simulink model "torqueBalancingTuning"  (Simulink 8.7)
settings: Solver=FixedStepDiscrete  StartTime=0.0  StopTime="CONFIG.SIMULATION_TIME "  FixedStep=CONFIG.Ts  RelTol=1e-3
InitFcn:
  | cd(fileparts(which(bdroot)));
  | initTorqueBalancing;
values from neighbouring files (symbols this model uses):
  baseToWorldRotationPort = ['/' WBT_modelName '/floatingBaseRotationMatrix:i']    [initTorqueBalancing.m]
  WBT_modelName = 'matlabTorqueBalancing'    [initTorqueBalancing.m]
undefined symbols (not defined in the file or in its folder): bVectorConstraints, CONFIG, ConstraintsMatrix, DiscIntNeverNeededParam, gain, references, reg, ROBOT_DOF, ROBOT_DOF_FOR_SIMULINK, sat, SM, sm, WBT_robotName
libraries: WBToolboxLibrary x171, simulink x11
(part 2 of 4)

== system torqueBalancingTuning/DesValues/Subsystem ==
  conn status 1 : Inport
  conn status 2 : Inport  Port=2
  conn status 3 : Inport  Port=3
  Compare To Zero3 : simulink/Logic and Bit Operations/Compare To Zero  relop=>  OutDataTypeStr=boolean
  Compare To Zero4 : simulink/Logic and Bit Operations/Compare To Zero  relop=>  OutDataTypeStr=boolean
  Compare To Zero5 : simulink/Logic and Bit Operations/Compare To Zero  relop=>  OutDataTypeStr=boolean
  Logical Operator : Logic  Inputs=3  AllPortsSameDT=off  OutDataTypeStr=boolean
  connection check : Outport
  wires:
  Logical Operator/1 -> connection check/1
  Compare To Zero4/1 -> Logical Operator/3
  conn status 1/1 -> Compare To Zero3/1
  Compare To Zero3/1 -> Logical Operator/1
  conn status 3/1 -> Compare To Zero4/1
  Compare To Zero5/1 -> Logical Operator/2
  conn status 2/1 -> Compare To Zero5/1

== system torqueBalancingTuning/Dump and visualize/ZMPs ==
  fDesQP : Inport
  Demux1 : Demux  Outputs=3
  Demux2 : Demux  Outputs=3
  Divide{4..7} (4 alike) : Product  Inputs=*/
  Gain3 : Gain  Gain=-1
  Gain4 : Gain  Gain=-1
  Mux : Mux  Inputs=2
  Mux1 : Mux  Inputs=2
  fz taux tauy Left : Selector  InputPortWidth=12  IndexOptions=Index vector (dialog)  Indices=[3 4 5]  OutputSizes=1
  fz taux tauy Right : Selector  InputPortWidth=12  IndexOptions=Index vector (dialog)  Indices=[9 10 11]  OutputSizes=1
  ZMP_LeftFoot : Outport
  ZMP_RightFoot : Outport  Port=2
  wires:
  fz taux tauy Left/1 -> Demux1/1
  Demux1/1 -> Divide4/2, Divide5/2
  Divide7/1 -> Gain4/1
  Divide4/1 -> Mux/2
  Divide5/1 -> Gain3/1
  fz taux tauy Right/1 -> Demux2/1
  Demux2/1 -> Divide6/2, Divide7/2
  fDesQP/1 -> fz taux tauy Left/1, fz taux tauy Right/1
  Gain3/1 -> Mux/1
  Mux/1 -> ZMP_LeftFoot/1
  Divide6/1 -> Mux1/2
  Gain4/1 -> Mux1/1
  Mux1/1 -> ZMP_RightFoot/1
  Demux1/2 -> Divide4/1  "tauxL"
  Demux1/3 -> Divide5/1  "tauyL"
  Demux2/2 -> Divide6/1  "tauxR"
  Demux2/3 -> Divide7/1  "tauyR"

== system torqueBalancingTuning/Dump and visualize/plotNorms ==
  qTile_LeftLeg : Inport
  qTile_RightLeg : Inport  Port=2
  state : Inport  Port=3
  Constant : Constant  Value=sm.joints.thresholdInContact
  Constant2 : Constant  Value=sm.joints.thresholdNotInContact
  Mux : Mux  Inputs=3
  Mux1 : Mux  Inputs=3
  norm : MATLAB Function  TreatAsAtomicUnit=on
  norm(qTilde) : Scope  NumInputPorts=3
  norm1 : MATLAB Function  TreatAsAtomicUnit=on
  wires:
  Constant/1 -> Mux1/2, Mux/2  "thresholdInContact"
  qTile_LeftLeg/1 -> norm1/1(u)
  qTile_RightLeg/1 -> norm/1(u)
  norm/1(normU) -> Mux1/1  "norm(qTilde_RightL)"
  norm1/1(normU) -> Mux/1  "norm(qTilde_LeftL)"
  Mux/1 -> norm(qTilde)/1
  Mux1/1 -> norm(qTilde)/2
  Constant2/1 -> Mux1/3, Mux/3  "thresholdNotInContact"
  state/1 -> norm(qTilde)/3

== system torqueBalancingTuning/controller_QP/QP ==
  LEFT_RIGHT_FOOT_IN_CONTACT : Inport
  HessianMatrixQP1Foot : Inport  Port=2
  gradientQP1Foot : Inport  Port=3
  ConstraintsMatrixQP1Foot : Inport  Port=4
  bVectorConstraintsQP1Foot : Inport  Port=5
  HessianMatrixQP2Feet : Inport  Port=6
  gradientQP2Feet : Inport  Port=7
  ConstraintsMatrixQP2Feet : Inport  Port=8
  bVectorConstraintsQp2Feet : Inport  Port=9
  state : Inport  Port=10
  Constant1 : Constant  Value=CONFIG.USE_QP_SOLVER
  Level-2 MATLAB S-Function : M-S-Function  FunctionName=QpBalancing
  Logical Operator1 : Logic  Operator=OR  AllPortsSameDT=off  OutDataTypeStr=boolean
  ON_GAZEBO 3 : Constant  Value=CONFIG.SCOPES.ALL
  ON_GAZEBO 4 : Constant  Value=CONFIG.SCOPES.QP
  QP two feet fails : Assertion  Commented=on
  Visualize eventual QP failures : Subsystem
  f0OneFoot : Outport
  f0TwoFeet : Outport  Port=2
  wires:
  Level-2 MATLAB S-Function/1 -> f0TwoFeet/1
  Level-2 MATLAB S-Function/2 -> Visualize eventual QP failures/1(exitFlagQP), QP two feet fails/1  "Exit flag QP two feet"
  HessianMatrixQP1Foot/1 -> Level-2 MATLAB S-Function/7
  gradientQP1Foot/1 -> Level-2 MATLAB S-Function/8
  ConstraintsMatrixQP1Foot/1 -> Level-2 MATLAB S-Function/9
  bVectorConstraintsQP1Foot/1 -> Level-2 MATLAB S-Function/10
  Level-2 MATLAB S-Function/3 -> f0OneFoot/1
  Logical Operator1/1 -> Visualize eventual QP failures/Enable
  state/1 -> Visualize eventual QP failures/2(state)
  LEFT_RIGHT_FOOT_IN_CONTACT/1 -> Level-2 MATLAB S-Function/1
  HessianMatrixQP2Feet/1 -> Level-2 MATLAB S-Function/2
  gradientQP2Feet/1 -> Level-2 MATLAB S-Function/3
  ConstraintsMatrixQP2Feet/1 -> Level-2 MATLAB S-Function/4
  bVectorConstraintsQp2Feet/1 -> Level-2 MATLAB S-Function/5
  Constant1/1 -> Level-2 MATLAB S-Function/6
  ON_GAZEBO 3/1 -> Logical Operator1/1
  ON_GAZEBO 4/1 -> Logical Operator1/2

== system torqueBalancingTuning/controller_QP/integralOf Hw1 ==
  qjDes : Inport
  qj : Inport  Port=2
  constraints : Inport  Port=3
  Centroidal Momentum : WBToolboxLibrary/wholeBodyModel/Dynamics/Centroidal Momentum  robotName=WBT_robotName  localName=WBT_modelName  wbiFile=WBT_wbiFilename  wbiList=WBT_wbiList
  Jacobian : WBToolboxLibrary/wholeBodyModel/Jacobians/Jacobian  frameName='l_sole'  robotName=WBT_robotName  localName=WBT_modelName  wbiFile=WBT_wbiFilename  wbiList=WBT_wbiList
  Jacobian1 : WBToolboxLibrary/wholeBodyModel/Jacobians/Jacobian  frameName='r_sole'  robotName=WBT_robotName  localName=WBT_modelName  wbiFile=WBT_wbiFilename  wbiList=WBT_wbiList
  MATLAB Function : MATLAB Function  TreatAsAtomicUnit=on
  Selector : Selector  InputPortWidth=6  IndexOptions=Index vector (dialog)  Indices=[4 5 6]  OutputSizes=1
  Sum : Sum  Inputs=|-+
  inertial : WBToolboxLibrary/Utilities/Yarp Read  portName=PORTS.IMU  signalSize=12  blocking=off  timestamp=off  autoconnect=on  errorOnConnection=on
  w_H_root_link4 : Subsystem  mask{link_name='l_sole'}
      mask prompts: link_name "link name"
      mask help:
      | This block evaluates the homogeneous transformation between the world and the root link, i.e. ^wH_b. It assumes that the link specified by the variable 'link_name' has a constant position
      | w.r.t. an inertial frame, but it can rotate arbitrarily. This rotation is retrived from the IMU sensor.
      mask Display:
      | str = strrep(link_name, '_','\_');
      | port_label('output',1,['{}^{',str '}H_{root}'],'texmode','on')
      | clear str;
      | 
      | port_label('input',1,'q_j','texmode','on')
      | 
      | port_label('input',2,'inertial','texmode','on')
  intHw : Outport
  wires:
  qjDes/1 -> Sum/1, Jacobian1/2, Jacobian/2, Centroidal Momentum/2, w_H_root_link4/1(qj)
  w_H_root_link4/1(w_H_root) -> Centroidal Momentum/1, Jacobian/1, Jacobian1/1
  qj/1 -> Sum/2
  Sum/1 -> Centroidal Momentum/4, MATLAB Function/1(qjErr)
  MATLAB Function/1(vbEquivalent) -> Centroidal Momentum/3
  Jacobian/1 -> MATLAB Function/2(JL)
  Centroidal Momentum/1 -> Selector/1
  Selector/1 -> intHw/1
  Jacobian1/1 -> MATLAB Function/3(JR)
  constraints/1 -> MATLAB Function/4(activeFeetConstraints)
  inertial/1 -> w_H_root_link4/2(inertial)

== system torqueBalancingTuning/controller_QP/xCom ==
  w_H_b : Inport
  qj : Inport  Port=2
  "CoM6D ->  CoMXYZ2" : Selector  NumberOfDimensions=2  InputPortWidth=7  IndexOptions=Index vector (dialog),Index vector (dialog)  Indices=[1 2 3],[4]  OutputSizes=1,1
  com : WBToolboxLibrary/wholeBodyModel/Kinematics/Forward Kinematics  frameName='com'  robotName=WBT_robotName  localName=WBT_modelName  wbiFile=WBT_wbiFilename  wbiList=WBT_wbiList
  xCom : Outport
  wires:
  qj/1 -> com/2
  "CoM6D ->  CoMXYZ2"/1 -> xCom/1
  com/1 -> "CoM6D ->  CoMXYZ2"/1
  w_H_b/1 -> com/1

== system torqueBalancingTuning/synchronizer/GAZEBO_SYNCHRONIZER ==
  Enable : EnablePort
  Simulator Synchronizer : WBToolboxLibrary/Utilities/Simulator Synchronizer  period=CONFIG.Ts  serverPortName='/clock/rpc'  clientPortName='/WBT_synchronizer/rpc:o'

== system torqueBalancingTuning/synchronizer/REAL_TIME_SYNC ==
  Enable : EnablePort
  Real Time Synchronizer : WBToolboxLibrary/Utilities/Real Time Synchronizer  period=CONFIG.Ts

== system torqueBalancingTuning/DesValues/Internal coordinator/nu ==
  qj : Inport
  w_H_b : Inport  Port=2
  "constraints " : Inport  Port=3
  Get Estimate : WBToolboxLibrary/wholeBodyStates/Get Estimate  estimateType=Joints Velocity  robotName=WBT_robotName  localName=WBT_modelName  wbiFile=WBT_wbiFilename  wbiList=WBT_wbiList
  Jacobian l_sole : WBToolboxLibrary/wholeBodyModel/Jacobians/Jacobian  frameName='l_sole'  robotName=WBT_robotName  localName=WBT_modelName  wbiFile=WBT_wbiFilename  wbiList=WBT_wbiList
  Jacobian r_sole : WBToolboxLibrary/wholeBodyModel/Jacobians/Jacobian  frameName='r_sole'  robotName=WBT_robotName  localName=WBT_modelName  wbiFile=WBT_wbiFilename  wbiList=WBT_wbiList
  MATLAB Function : MATLAB Function  TreatAsAtomicUnit=on
  Mux : Mux  Inputs=2
  vb + Dqj : Outport
  wires:
  Get Estimate/1 -> MATLAB Function/4(qD), Mux/2
  Mux/1 -> vb + Dqj/1
  Jacobian r_sole/1 -> MATLAB Function/2(JcRightFoot)
  "constraints "/1 -> MATLAB Function/3(activeFeetConstraints)
  MATLAB Function/1(y) -> Mux/1
  Jacobian l_sole/1 -> MATLAB Function/1(JcLeftFoot)
  qj/1 -> Jacobian r_sole/2, Jacobian l_sole/2
  w_H_b/1 -> Jacobian r_sole/1, Jacobian l_sole/1

== system torqueBalancingTuning/DesValues/Internal coordinator/refGen ==
  xCom(0) : Inport
  qj(0) : Inport  Port=2
  Enable : EnablePort
  Clock1 : Clock
  refGenFCN : MATLAB Function  TreatAsAtomicUnit=on
  qDes : Outport
  CoMrefs : Outport  Port=2
  wires:
  refGenFCN/2(desired_x_dx_ddx_CoM) -> CoMrefs/1
  xCom(0)/1 -> refGenFCN/1(xCom0)
  Clock1/1 -> refGenFCN/3(t)
  qj(0)/1 -> refGenFCN/2(q0)
  refGenFCN/1(qDes) -> qDes/1

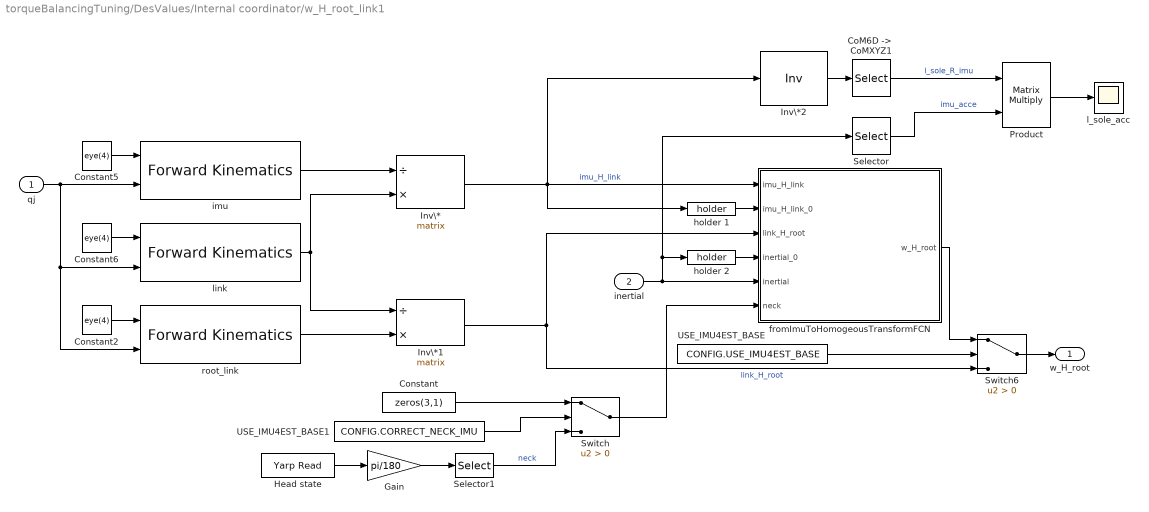
== system torqueBalancingTuning/DesValues/Internal coordinator/w_H_root_link1 ==
  qj : Inport
  inertial : Inport  Port=2
  "CoM6D ->  CoMXYZ1" : Selector  NumberOfDimensions=2  InputPortWidth=7  IndexOptions=Index vector (dialog),Index vector (dialog)  Indices=[1 2 3],[1 2 3]  OutputSizes=1,1
  Constant : Constant  Value=zeros(3,1)
  Constant2 : Constant  Value=eye(4)
  Constant5 : Constant  Value=eye(4)
  Constant6 : Constant  Value=eye(4)
  Gain : Gain  Gain=pi/180
  Head state : WBToolboxLibrary/Utilities/Yarp Read  portName=[WBT_robotName, '/head/state:o']  signalSize=6  blocking=off  timestamp=off  autoconnect=on  errorOnConnection=off
  Inv\* : Product  Inputs=/*  Multiplication=Matrix(*)
  Inv\*1 : Product  Inputs=/*  Multiplication=Matrix(*)
  Inv\*2 : Product  Inputs=/  Multiplication=Matrix(*)
  Product : Product  Multiplication=Matrix(*)
  Selector : Selector  InputPortWidth=12  IndexOptions=Index vector (dialog)  Indices=[4 5 6 ]  OutputSizes=1
  Selector1 : Selector  InputPortWidth=6  IndexOptions=Index vector (dialog)  Indices=[1:3]  OutputSizes=1
  Switch : Switch  Criteria=u2 > Threshold
  Switch6 : Switch  Criteria=u2 > Threshold
  USE_IMU4EST_BASE : Constant  Value=CONFIG.USE_IMU4EST_BASE
  USE_IMU4EST_BASE1 : Constant  Value=CONFIG.CORRECT_NECK_IMU
  fromImuToHomogeousTransformFCN : MATLAB Function  TreatAsAtomicUnit=on
  holder 1 : WBToolboxLibrary/Utilities/holder 
  holder 2 : WBToolboxLibrary/Utilities/holder 
  imu : WBToolboxLibrary/wholeBodyModel/Kinematics/Forward Kinematics  frameName='imu_frame'  robotName=WBT_robotName  localName=WBT_modelName  wbiFile=WBT_wbiFilename  wbiList=WBT_wbiList
  l_sole_acc : Scope
  link : WBToolboxLibrary/wholeBodyModel/Kinematics/Forward Kinematics  frameName=link_name  robotName=WBT_robotName  localName=WBT_modelName  wbiFile=WBT_wbiFilename  wbiList=WBT_wbiList
  root_link : WBToolboxLibrary/wholeBodyModel/Kinematics/Forward Kinematics  frameName='root_link'  robotName=WBT_robotName  localName=WBT_modelName  wbiFile=WBT_wbiFilename  wbiList=WBT_wbiList
  w_H_root : Outport
  wires:
  Constant5/1 -> imu/1
  Inv\*/1 -> Inv\*2/1, holder 1/1, fromImuToHomogeousTransformFCN/1(imu_H_link)  "imu_H_link"
  imu/1 -> Inv\*/1
  Constant6/1 -> link/1
  Inv\*1/1 -> Switch6/3, fromImuToHomogeousTransformFCN/3(link_H_root)  "link_H_root"
  link/1 -> Inv\*/2, Inv\*1/1
  inertial/1 -> Selector/1, holder 2/1, fromImuToHomogeousTransformFCN/5(inertial)
  Switch6/1 -> w_H_root/1
  USE_IMU4EST_BASE/1 -> Switch6/2
  fromImuToHomogeousTransformFCN/1(w_H_root) -> Switch6/1
  Constant2/1 -> root_link/1
  qj/1 -> root_link/2, link/2, imu/2
  root_link/1 -> Inv\*1/2
  holder 1/1 -> fromImuToHomogeousTransformFCN/2(imu_H_link_0)
  holder 2/1 -> fromImuToHomogeousTransformFCN/4(inertial_0)
  Inv\*2/1 -> "CoM6D ->  CoMXYZ1"/1
  "CoM6D ->  CoMXYZ1"/1 -> Product/1  "l_sole_R_imu"
  Selector/1 -> Product/2  "imu_acce"
  Product/1 -> l_sole_acc/1
  Head state/1 -> Gain/1
  Selector1/1 -> Switch/3  "neck"
  Constant/1 -> Switch/1
  USE_IMU4EST_BASE1/1 -> Switch/2
  Switch/1 -> fromImuToHomogeousTransformFCN/6(neck)
  Gain/1 -> Selector1/1

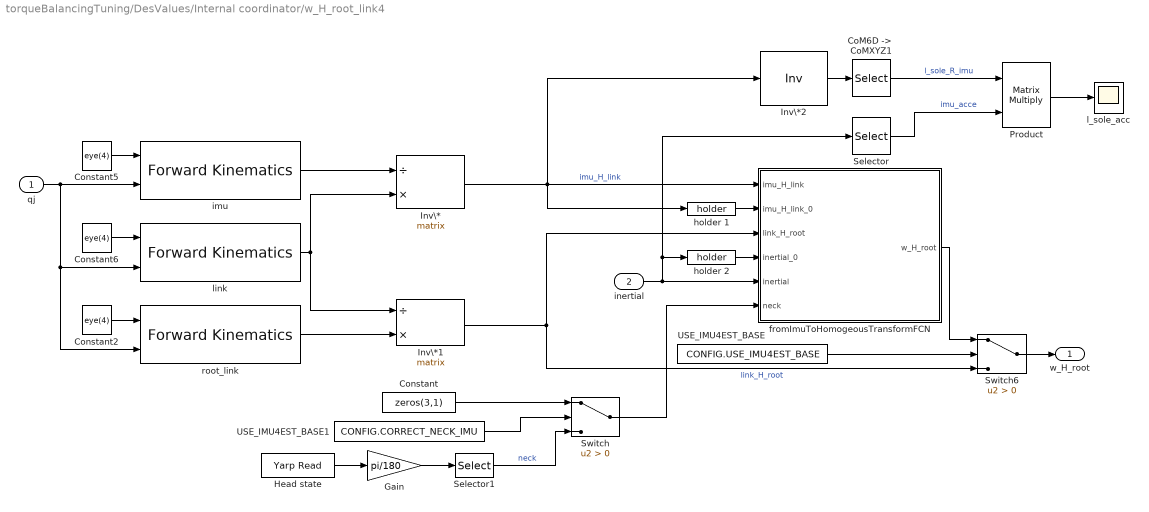
== system torqueBalancingTuning/DesValues/Internal coordinator/w_H_root_link4 ==
  qj : Inport
  inertial : Inport  Port=2
  "CoM6D ->  CoMXYZ1" : Selector  NumberOfDimensions=2  InputPortWidth=7  IndexOptions=Index vector (dialog),Index vector (dialog)  Indices=[1 2 3],[1 2 3]  OutputSizes=1,1
  Constant : Constant  Value=zeros(3,1)
  Constant2 : Constant  Value=eye(4)
  Constant5 : Constant  Value=eye(4)
  Constant6 : Constant  Value=eye(4)
  Gain : Gain  Gain=pi/180
  Head state : WBToolboxLibrary/Utilities/Yarp Read  portName=[WBT_robotName, '/head/state:o']  signalSize=6  blocking=off  timestamp=off  autoconnect=on  errorOnConnection=off
  Inv\* : Product  Inputs=/*  Multiplication=Matrix(*)
  Inv\*1 : Product  Inputs=/*  Multiplication=Matrix(*)
  Inv\*2 : Product  Inputs=/  Multiplication=Matrix(*)
  Product : Product  Multiplication=Matrix(*)
  Selector : Selector  InputPortWidth=12  IndexOptions=Index vector (dialog)  Indices=[4 5 6 ]  OutputSizes=1
  Selector1 : Selector  InputPortWidth=6  IndexOptions=Index vector (dialog)  Indices=[1:3]  OutputSizes=1
  Switch : Switch  Criteria=u2 > Threshold
  Switch6 : Switch  Criteria=u2 > Threshold
  USE_IMU4EST_BASE : Constant  Value=CONFIG.USE_IMU4EST_BASE
  USE_IMU4EST_BASE1 : Constant  Value=CONFIG.CORRECT_NECK_IMU
  fromImuToHomogeousTransformFCN : MATLAB Function  TreatAsAtomicUnit=on
  holder 1 : WBToolboxLibrary/Utilities/holder 
  holder 2 : WBToolboxLibrary/Utilities/holder 
  imu : WBToolboxLibrary/wholeBodyModel/Kinematics/Forward Kinematics  frameName='imu_frame'  robotName=WBT_robotName  localName=WBT_modelName  wbiFile=WBT_wbiFilename  wbiList=WBT_wbiList
  l_sole_acc : Scope
  link : WBToolboxLibrary/wholeBodyModel/Kinematics/Forward Kinematics  frameName=link_name  robotName=WBT_robotName  localName=WBT_modelName  wbiFile=WBT_wbiFilename  wbiList=WBT_wbiList
  root_link : WBToolboxLibrary/wholeBodyModel/Kinematics/Forward Kinematics  frameName='root_link'  robotName=WBT_robotName  localName=WBT_modelName  wbiFile=WBT_wbiFilename  wbiList=WBT_wbiList
  w_H_root : Outport
  wires:
  Constant5/1 -> imu/1
  Inv\*/1 -> Inv\*2/1, holder 1/1, fromImuToHomogeousTransformFCN/1(imu_H_link)  "imu_H_link"
  imu/1 -> Inv\*/1
  Constant6/1 -> link/1
  Inv\*1/1 -> Switch6/3, fromImuToHomogeousTransformFCN/3(link_H_root)  "link_H_root"
  link/1 -> Inv\*/2, Inv\*1/1
  inertial/1 -> Selector/1, holder 2/1, fromImuToHomogeousTransformFCN/5(inertial)
  Switch6/1 -> w_H_root/1
  USE_IMU4EST_BASE/1 -> Switch6/2
  fromImuToHomogeousTransformFCN/1(w_H_root) -> Switch6/1
  Constant2/1 -> root_link/1
  qj/1 -> root_link/2, link/2, imu/2
  root_link/1 -> Inv\*1/2
  holder 1/1 -> fromImuToHomogeousTransformFCN/2(imu_H_link_0)
  holder 2/1 -> fromImuToHomogeousTransformFCN/4(inertial_0)
  Inv\*2/1 -> "CoM6D ->  CoMXYZ1"/1
  "CoM6D ->  CoMXYZ1"/1 -> Product/1  "l_sole_R_imu"
  Selector/1 -> Product/2  "imu_acce"
  Product/1 -> l_sole_acc/1
  Head state/1 -> Gain/1
  Selector1/1 -> Switch/3  "neck"
  Constant/1 -> Switch/1
  USE_IMU4EST_BASE1/1 -> Switch/2
  Switch/1 -> fromImuToHomogeousTransformFCN/6(neck)
  Gain/1 -> Selector1/1

== system torqueBalancingTuning/DesValues/Internal coordinator/xCom ==
  w_H_b : Inport
  qj : Inport  Port=2
  "CoM6D ->  CoMXYZ2" : Selector  NumberOfDimensions=2  InputPortWidth=7  IndexOptions=Index vector (dialog),Index vector (dialog)  Indices=[1 2 3],[4]  OutputSizes=1,1
  com : WBToolboxLibrary/wholeBodyModel/Kinematics/Forward Kinematics  frameName='com'  robotName=WBT_robotName  localName=WBT_modelName  wbiFile=WBT_wbiFilename  wbiList=WBT_wbiList
  xCom : Outport
  wires:
  qj/1 -> com/2
  "CoM6D ->  CoMXYZ2"/1 -> xCom/1
  com/1 -> "CoM6D ->  CoMXYZ2"/1
  w_H_b/1 -> com/1

== system torqueBalancingTuning/DesValues/Internal coordinator/xCom1 ==
  w_H_b : Inport
  qj : Inport  Port=2
  "CoM6D ->  CoMXYZ2" : Selector  NumberOfDimensions=2  InputPortWidth=7  IndexOptions=Index vector (dialog),Index vector (dialog)  Indices=[1 2 3],[4]  OutputSizes=1,1
  com : WBToolboxLibrary/wholeBodyModel/Kinematics/Forward Kinematics  frameName='com'  robotName=WBT_robotName  localName=WBT_modelName  wbiFile=WBT_wbiFilename  wbiList=WBT_wbiList
  xCom : Outport
  wires:
  qj/1 -> com/2
  "CoM6D ->  CoMXYZ2"/1 -> xCom/1
  com/1 -> "CoM6D ->  CoMXYZ2"/1
  w_H_b/1 -> com/1

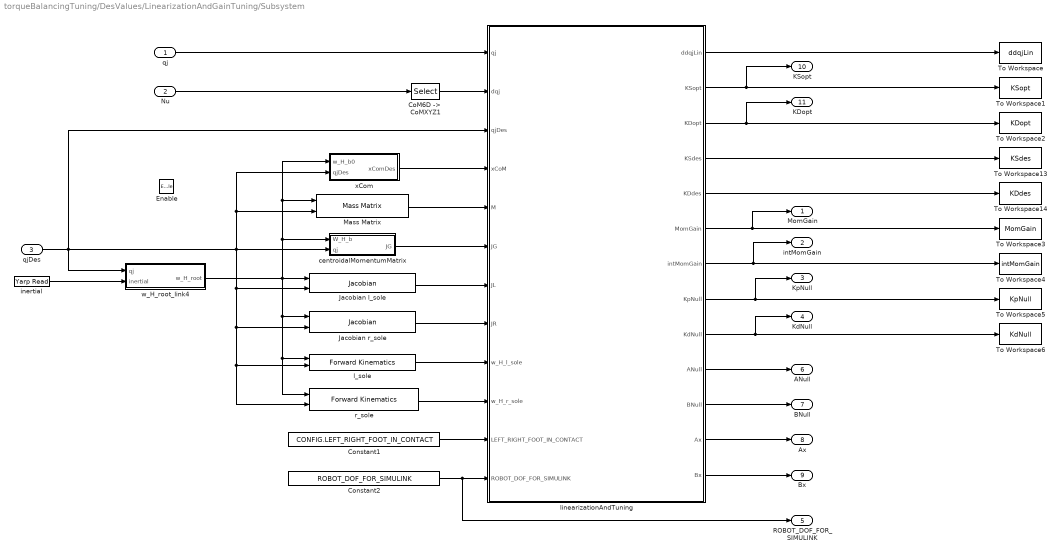
== system torqueBalancingTuning/DesValues/LinearizationAndGainTuning/Subsystem ==
  qj : Inport
  Nu : Inport  Port=2
  qjDes : Inport  Port=3
  Enable : EnablePort
  "CoM6D ->  CoMXYZ1" : Selector  InputPortWidth=6+ROBOT_DOF  IndexOptions=Index vector (dialog)  Indices=[7:6+ROBOT_DOF]  OutputSizes=1
  Constant1 : Constant  Value=CONFIG.LEFT_RIGHT_FOOT_IN_CONTACT
  Constant2 : Constant  Value=ROBOT_DOF_FOR_SIMULINK
  Jacobian l_sole : WBToolboxLibrary/wholeBodyModel/Jacobians/Jacobian  frameName='l_sole'  robotName=WBT_robotName  localName=WBT_modelName  wbiFile=WBT_wbiFilename  wbiList=WBT_wbiList
  Jacobian r_sole : WBToolboxLibrary/wholeBodyModel/Jacobians/Jacobian  frameName='r_sole'  robotName=WBT_robotName  localName=WBT_modelName  wbiFile=WBT_wbiFilename  wbiList=WBT_wbiList
  Mass Matrix : WBToolboxLibrary/wholeBodyModel/Dynamics/Mass Matrix  robotName=WBT_robotName  localName=WBT_modelName  wbiFile=WBT_wbiFilename  wbiList=WBT_wbiList
  To Workspace : ToWorkspace  VariableName=ddqjLin  SaveFormat=Structure With Time  SampleTime=-1
  To Workspace1 : ToWorkspace  VariableName=KSopt  SaveFormat=Structure With Time  SampleTime=-1
  To Workspace13 : ToWorkspace  VariableName=KSdes  SaveFormat=Structure With Time  SampleTime=-1
  To Workspace14 : ToWorkspace  VariableName=KDdes  SaveFormat=Structure With Time  SampleTime=-1
  To Workspace2 : ToWorkspace  VariableName=KDopt  SaveFormat=Structure With Time  SampleTime=-1
  To Workspace3 : ToWorkspace  VariableName=MomGain  SaveFormat=Structure With Time  SampleTime=-1
  To Workspace4 : ToWorkspace  VariableName=intMomGain  SaveFormat=Structure With Time  SampleTime=-1
  To Workspace5 : ToWorkspace  VariableName=KpNull  SaveFormat=Structure With Time  SampleTime=-1
  To Workspace6 : ToWorkspace  VariableName=KdNull  SaveFormat=Structure With Time  SampleTime=-1
  centroidalMomentumMatrix : Subsystem
  inertial : WBToolboxLibrary/Utilities/Yarp Read  portName=PORTS.IMU  signalSize=12  blocking=off  timestamp=off  autoconnect=on  errorOnConnection=on
  l_sole : WBToolboxLibrary/wholeBodyModel/Kinematics/Forward Kinematics  frameName='l_sole'  robotName=WBT_robotName  localName=WBT_modelName  wbiFile=WBT_wbiFilename  wbiList=WBT_wbiList
  linearizationAndTuning : MATLAB Function  TreatAsAtomicUnit=on
  r_sole : WBToolboxLibrary/wholeBodyModel/Kinematics/Forward Kinematics  frameName='r_sole'  robotName=WBT_robotName  localName=WBT_modelName  wbiFile=WBT_wbiFilename  wbiList=WBT_wbiList
  w_H_root_link4 : Subsystem  mask{link_name='l_sole'}
      mask prompts: link_name "link name"
      mask help:
      | This block evaluates the homogeneous transformation between the world and the root link, i.e. ^wH_b. It assumes that the link specified by the variable 'link_name' has a constant position
      | w.r.t. an inertial frame, but it can rotate arbitrarily. This rotation is retrived from the IMU sensor.
      mask Display:
      | str = strrep(link_name, '_','\_');
      | port_label('output',1,['{}^{',str '}H_{root}'],'texmode','on')
      | clear str;
      | 
      | port_label('input',1,'q_j','texmode','on')
      | 
      | port_label('input',2,'inertial','texmode','on')
  xCom : Subsystem
  MomGain : Outport
  intMomGain : Outport  Port=2
  KpNull : Outport  Port=3
  KdNull : Outport  Port=4
  "ROBOT_DOF_FOR_SIMULINK " : Outport  Port=5
  ANull : Outport  Port=6
  BNull : Outport  Port=7
  Ax : Outport  Port=8
  Bx : Outport  Port=9
  KSopt : Outport  Port=10
  KDopt : Outport  Port=11
  wires:
  w_H_root_link4/1(w_H_root) -> Jacobian r_sole/1, l_sole/1, r_sole/1, xCom/1(w_H_b0), Mass Matrix/1, centroidalMomentumMatrix/1(W_H_b), Jacobian l_sole/1
  xCom/1(xComDes) -> linearizationAndTuning/4(xCoM)
  Mass Matrix/1 -> linearizationAndTuning/5(M)
  Constant1/1 -> linearizationAndTuning/11(LEFT_RIGHT_FOOT_IN_CONTACT)
  Jacobian r_sole/1 -> linearizationAndTuning/8(JR)
  Jacobian l_sole/1 -> linearizationAndTuning/7(JL)
  l_sole/1 -> linearizationAndTuning/9(w_H_l_sole)
  r_sole/1 -> linearizationAndTuning/10(w_H_r_sole)
  Constant2/1 -> "ROBOT_DOF_FOR_SIMULINK "/1, linearizationAndTuning/12(ROBOT_DOF_FOR_SIMULINK)
  centroidalMomentumMatrix/1(JG) -> linearizationAndTuning/6(JG)
  qjDes/1 -> xCom/2(qjDes), Mass Matrix/2, centroidalMomentumMatrix/2(qj), Jacobian l_sole/2, r_sole/2, l_sole/2, Jacobian r_sole/2, linearizationAndTuning/3(qjDes), w_H_root_link4/1(qj)
  qj/1 -> linearizationAndTuning/1(qj)
  Nu/1 -> "CoM6D ->  CoMXYZ1"/1
  "CoM6D ->  CoMXYZ1"/1 -> linearizationAndTuning/2(dqj)
  linearizationAndTuning/1(ddqjLin) -> To Workspace/1
  linearizationAndTuning/2(KSopt) -> KSopt/1, To Workspace1/1
  linearizationAndTuning/3(KDopt) -> KDopt/1, To Workspace2/1
  inertial/1 -> w_H_root_link4/2(inertial)
  linearizationAndTuning/6(MomGain) -> To Workspace3/1, MomGain/1
  linearizationAndTuning/4(KSdes) -> To Workspace13/1
  linearizationAndTuning/5(KDdes) -> To Workspace14/1
  linearizationAndTuning/7(intMomGain) -> To Workspace4/1, intMomGain/1
  linearizationAndTuning/8(KpNull) -> To Workspace5/1, KpNull/1
  linearizationAndTuning/9(KdNull) -> To Workspace6/1, KdNull/1
  linearizationAndTuning/10(ANull) -> ANull/1
  linearizationAndTuning/11(BNull) -> BNull/1
  linearizationAndTuning/12(Ax) -> Ax/1
  linearizationAndTuning/13(Bx) -> Bx/1

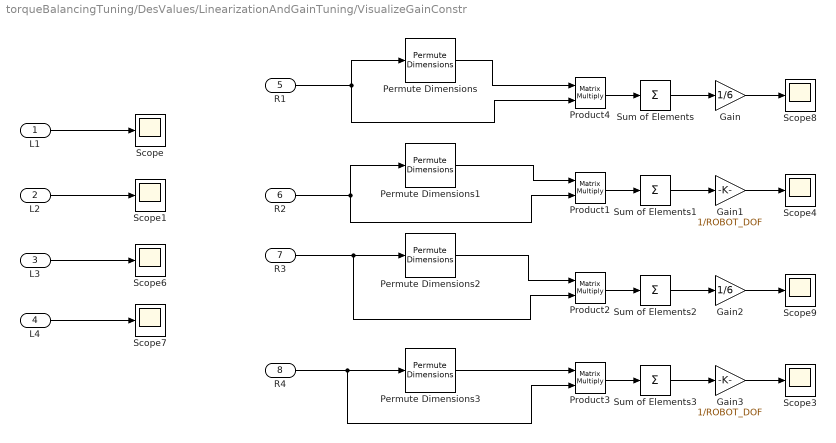
== system torqueBalancingTuning/DesValues/LinearizationAndGainTuning/VisualizeGainConstr ==
  L1 : Inport
  L2 : Inport  Port=2
  L3 : Inport  Port=3
  L4 : Inport  Port=4
  R1 : Inport  Port=5
  R2 : Inport  Port=6
  R3 : Inport  Port=7
  R4 : Inport  Port=8
  Gain : Gain  Gain=1/6
  Gain1 : Gain  Gain=1/ROBOT_DOF
  Gain2 : Gain  Gain=1/6
  Gain3 : Gain  Gain=1/ROBOT_DOF
  Permute Dimensions{,1..3} (4 alike) : PermuteDimensions
  Product{1..4} (4 alike) : Product  Multiplication=Matrix(*)
  Scope{,1,3..4,6..9} (8 alike) : Scope
  Sum of Elements{,1..3} (4 alike) : Sum  Inputs=+
  wires:
  L2/1 -> Scope1/1
  R3/1 -> Product2/2, Permute Dimensions2/1
  L3/1 -> Scope6/1
  L4/1 -> Scope7/1
  L1/1 -> Scope/1
  R1/1 -> Product4/2, Permute Dimensions/1
  R2/1 -> Product1/2, Permute Dimensions1/1
  R4/1 -> Product3/2, Permute Dimensions3/1
  Product4/1 -> Sum of Elements/1
  Product1/1 -> Sum of Elements1/1
  Product2/1 -> Sum of Elements2/1
  Product3/1 -> Sum of Elements3/1
  Permute Dimensions/1 -> Product4/1
  Permute Dimensions1/1 -> Product1/1
  Permute Dimensions2/1 -> Product2/1
  Permute Dimensions3/1 -> Product3/1
  Sum of Elements/1 -> Gain/1
  Sum of Elements1/1 -> Gain1/1
  Sum of Elements2/1 -> Gain2/1
  Sum of Elements3/1 -> Gain3/1
  Gain/1 -> Scope8/1
  Gain1/1 -> Scope4/1
  Gain2/1 -> Scope9/1
  Gain3/1 -> Scope3/1

== system torqueBalancingTuning/DesValues/State Machine/Visualise extrnal wrenches   ==
  wL_WBDT : Inport
  wR_WBDT : Inport  Port=2
  Enable : EnablePort
  Constant : Constant  Value=sm.wrench.thresholdContactOn
  Constant2 : Constant  Value=sm.wrench.thresholdContactOff
  left foot ext wrench : Scope  NumInputPorts=3
  right foot ext wrench : Scope  NumInputPorts=3
  wires:
  Constant/1 -> left foot ext wrench/2, right foot ext wrench/2  "thresholdContactOn"
  wR_WBDT/1 -> right foot ext wrench/1  "wR_WBDT"
  wL_WBDT/1 -> left foot ext wrench/1  "wL_WBDT"
  Constant2/1 -> left foot ext wrench/3, right foot ext wrench/3  "thresholdContactOff"

== system torqueBalancingTuning/DesValues/State Machine/nu ==
  qj : Inport
  w_H_b : Inport  Port=2
  "constraints " : Inport  Port=3
  Get Estimate : WBToolboxLibrary/wholeBodyStates/Get Estimate  estimateType=Joints Velocity  robotName=WBT_robotName  localName=WBT_modelName  wbiFile=WBT_wbiFilename  wbiList=WBT_wbiList
  Jacobian l_sole : WBToolboxLibrary/wholeBodyModel/Jacobians/Jacobian  frameName='l_sole'  robotName=WBT_robotName  localName=WBT_modelName  wbiFile=WBT_wbiFilename  wbiList=WBT_wbiList
  Jacobian r_sole : WBToolboxLibrary/wholeBodyModel/Jacobians/Jacobian  frameName='r_sole'  robotName=WBT_robotName  localName=WBT_modelName  wbiFile=WBT_wbiFilename  wbiList=WBT_wbiList
  MATLAB Function : MATLAB Function  TreatAsAtomicUnit=on
  Mux : Mux  Inputs=2
  vb + Dqj : Outport
  wires:
  Get Estimate/1 -> MATLAB Function/4(qD), Mux/2
  Mux/1 -> vb + Dqj/1
  Jacobian r_sole/1 -> MATLAB Function/2(JcRightFoot)
  "constraints "/1 -> MATLAB Function/3(activeFeetConstraints)
  MATLAB Function/1(y) -> Mux/1
  Jacobian l_sole/1 -> MATLAB Function/1(JcLeftFoot)
  qj/1 -> Jacobian r_sole/2, Jacobian l_sole/2
  w_H_b/1 -> Jacobian r_sole/1, Jacobian l_sole/1

== system torqueBalancingTuning/DesValues/State Machine/visualise inertial ==
  jointAngles : Inport
  inertial : Inport  Port=2
  Enable : EnablePort
  Inv\* : Product  Inputs=/*  Multiplication=Matrix(*)
  Inv\*1 : Product  Inputs=/*  Multiplication=Matrix(*)
  Visualize hom transf1 : Subsystem
  Visualize hom transf2 : Subsystem
  Visualize hom transf3 : Subsystem
  Visualize hom transf4 : Subsystem
  Visualize hom transf5 : Subsystem
  Visualize hom transf6 : Subsystem
  "inertial -> rpy" : Selector  InputPortWidth=12  IndexOptions=Index vector (dialog)  Indices=[1 2 3]  OutputSizes=1
  l_sole_H_root_link2 : Subsystem  mask{link_name='l_sole'}
  l_sole_H_root_link3 : Subsystem  mask{link_name='r_sole'}
  rpy : Scope
  w_H_root_link1 : Subsystem  mask{link_name='r_sole'}
      mask prompts: link_name "link name"
      mask help:
      | This block evaluates the homogeneous transformation between the world and the root link, i.e. ^wH_b. It assumes that the link specified by the variable 'link_name' has a constant position
      | w.r.t. an inertial frame, but it can rotate arbitrarily. This rotation is retrived from the IMU sensor.
      mask Display:
      | str = strrep(link_name, '_','\_');
      | port_label('output',1,['{}^{',str '}H_{root}'],'texmode','on')
      | clear str;
      | 
      | port_label('input',1,'q_j','texmode','on')
      | 
      | port_label('input',2,'inertial','texmode','on')
  w_H_root_link4 : Subsystem  mask{link_name='l_sole'}
      mask prompts: link_name "link name"
      mask help:
      | This block evaluates the homogeneous transformation between the world and the root link, i.e. ^wH_b. It assumes that the link specified by the variable 'link_name' has a constant position
      | w.r.t. an inertial frame, but it can rotate arbitrarily. This rotation is retrived from the IMU sensor.
      mask Display:
      | str = strrep(link_name, '_','\_');
      | port_label('output',1,['{}^{',str '}H_{root}'],'texmode','on')
      | clear str;
      | 
      | port_label('input',1,'q_j','texmode','on')
      | 
      | port_label('input',2,'inertial','texmode','on')
  wires:
  inertial/1 -> "inertial -> rpy"/1, w_H_root_link1/2(inertial), w_H_root_link4/2(inertial)
  jointAngles/1 -> l_sole_H_root_link2/1(qj), w_H_root_link4/1(qj), w_H_root_link1/1(qj), l_sole_H_root_link3/1(qj)
  l_sole_H_root_link2/1(link_name_H_root_link) -> Visualize hom transf6/1(H), Inv\*/1  "l_sole_H_root_link"
  Inv\*/1 -> Visualize hom transf5/1(H)
  w_H_root_link4/1(w_H_root) -> Visualize hom transf4/1(H), Inv\*/2
  "inertial -> rpy"/1 -> rpy/1
  l_sole_H_root_link3/1(link_name_H_root_link) -> Visualize hom transf2/1(H), Inv\*1/1  "r_sole_H_root_link"
  Inv\*1/1 -> Visualize hom transf1/1(H)
  w_H_root_link1/1(w_H_root) -> Visualize hom transf3/1(H), Inv\*1/2

== system torqueBalancingTuning/DesValues/State Machine/w_H_root_link1 ==
  qj : Inport
  inertial : Inport  Port=2
  "CoM6D ->  CoMXYZ1" : Selector  NumberOfDimensions=2  InputPortWidth=7  IndexOptions=Index vector (dialog),Index vector (dialog)  Indices=[1 2 3],[1 2 3]  OutputSizes=1,1
  Constant : Constant  Value=zeros(3,1)
  Constant2 : Constant  Value=eye(4)
  Constant5 : Constant  Value=eye(4)
  Constant6 : Constant  Value=eye(4)
  Gain : Gain  Gain=pi/180
  Head state : WBToolboxLibrary/Utilities/Yarp Read  portName=[WBT_robotName, '/head/state:o']  signalSize=6  blocking=off  timestamp=off  autoconnect=on  errorOnConnection=off
  Inv\* : Product  Inputs=/*  Multiplication=Matrix(*)
  Inv\*1 : Product  Inputs=/*  Multiplication=Matrix(*)
  Inv\*2 : Product  Inputs=/  Multiplication=Matrix(*)
  Product : Product  Multiplication=Matrix(*)
  Selector : Selector  InputPortWidth=12  IndexOptions=Index vector (dialog)  Indices=[4 5 6 ]  OutputSizes=1
  Selector1 : Selector  InputPortWidth=6  IndexOptions=Index vector (dialog)  Indices=[1:3]  OutputSizes=1
  Switch : Switch  Criteria=u2 > Threshold
  Switch6 : Switch  Criteria=u2 > Threshold
  USE_IMU4EST_BASE : Constant  Value=CONFIG.USE_IMU4EST_BASE
  USE_IMU4EST_BASE1 : Constant  Value=CONFIG.CORRECT_NECK_IMU
  fromImuToHomogeousTransformFCN : MATLAB Function  TreatAsAtomicUnit=on
  holder 1 : WBToolboxLibrary/Utilities/holder 
  holder 2 : WBToolboxLibrary/Utilities/holder 
  imu : WBToolboxLibrary/wholeBodyModel/Kinematics/Forward Kinematics  frameName='imu_frame'  robotName=WBT_robotName  localName=WBT_modelName  wbiFile=WBT_wbiFilename  wbiList=WBT_wbiList
  l_sole_acc : Scope
  link : WBToolboxLibrary/wholeBodyModel/Kinematics/Forward Kinematics  frameName=link_name  robotName=WBT_robotName  localName=WBT_modelName  wbiFile=WBT_wbiFilename  wbiList=WBT_wbiList
  root_link : WBToolboxLibrary/wholeBodyModel/Kinematics/Forward Kinematics  frameName='root_link'  robotName=WBT_robotName  localName=WBT_modelName  wbiFile=WBT_wbiFilename  wbiList=WBT_wbiList
  w_H_root : Outport
  wires:
  Constant5/1 -> imu/1
  Inv\*/1 -> Inv\*2/1, holder 1/1, fromImuToHomogeousTransformFCN/1(imu_H_link)  "imu_H_link"
  imu/1 -> Inv\*/1
  Constant6/1 -> link/1
  Inv\*1/1 -> Switch6/3, fromImuToHomogeousTransformFCN/3(link_H_root)  "link_H_root"
  link/1 -> Inv\*/2, Inv\*1/1
  inertial/1 -> Selector/1, holder 2/1, fromImuToHomogeousTransformFCN/5(inertial)
  Switch6/1 -> w_H_root/1
  USE_IMU4EST_BASE/1 -> Switch6/2
  fromImuToHomogeousTransformFCN/1(w_H_root) -> Switch6/1
  Constant2/1 -> root_link/1
  qj/1 -> root_link/2, link/2, imu/2
  root_link/1 -> Inv\*1/2
  holder 1/1 -> fromImuToHomogeousTransformFCN/2(imu_H_link_0)
  holder 2/1 -> fromImuToHomogeousTransformFCN/4(inertial_0)
  Inv\*2/1 -> "CoM6D ->  CoMXYZ1"/1
  "CoM6D ->  CoMXYZ1"/1 -> Product/1  "l_sole_R_imu"
  Selector/1 -> Product/2  "imu_acce"
  Product/1 -> l_sole_acc/1
  Head state/1 -> Gain/1
  Selector1/1 -> Switch/1  "neck"
  USE_IMU4EST_BASE1/1 -> Switch/2
  Switch/1 -> fromImuToHomogeousTransformFCN/6(neck)
  Gain/1 -> Selector1/1
  Constant/1 -> Switch/3

== system torqueBalancingTuning/DesValues/State Machine/w_H_root_link4 ==
  qj : Inport
  inertial : Inport  Port=2
  "CoM6D ->  CoMXYZ1" : Selector  NumberOfDimensions=2  InputPortWidth=7  IndexOptions=Index vector (dialog),Index vector (dialog)  Indices=[1 2 3],[1 2 3]  OutputSizes=1,1
  Constant : Constant  Value=zeros(3,1)
  Constant2 : Constant  Value=eye(4)
  Constant5 : Constant  Value=eye(4)
  Constant6 : Constant  Value=eye(4)
  Gain : Gain  Gain=pi/180
  Head state : WBToolboxLibrary/Utilities/Yarp Read  portName=[WBT_robotName, '/head/state:o']  signalSize=6  blocking=off  timestamp=off  autoconnect=on  errorOnConnection=off
  Inv\* : Product  Inputs=/*  Multiplication=Matrix(*)
  Inv\*1 : Product  Inputs=/*  Multiplication=Matrix(*)
  Inv\*2 : Product  Inputs=/  Multiplication=Matrix(*)
  Product : Product  Multiplication=Matrix(*)
  Selector : Selector  InputPortWidth=12  IndexOptions=Index vector (dialog)  Indices=[4 5 6 ]  OutputSizes=1
  Selector1 : Selector  InputPortWidth=6  IndexOptions=Index vector (dialog)  Indices=[1:3]  OutputSizes=1
  Switch : Switch  Criteria=u2 > Threshold
  Switch6 : Switch  Criteria=u2 > Threshold
  USE_IMU4EST_BASE : Constant  Value=CONFIG.USE_IMU4EST_BASE
  USE_IMU4EST_BASE1 : Constant  Value=CONFIG.CORRECT_NECK_IMU
  fromImuToHomogeousTransformFCN : MATLAB Function  TreatAsAtomicUnit=on
  holder 1 : WBToolboxLibrary/Utilities/holder 
  holder 2 : WBToolboxLibrary/Utilities/holder 
  imu : WBToolboxLibrary/wholeBodyModel/Kinematics/Forward Kinematics  frameName='imu_frame'  robotName=WBT_robotName  localName=WBT_modelName  wbiFile=WBT_wbiFilename  wbiList=WBT_wbiList
  l_sole_acc : Scope
  link : WBToolboxLibrary/wholeBodyModel/Kinematics/Forward Kinematics  frameName=link_name  robotName=WBT_robotName  localName=WBT_modelName  wbiFile=WBT_wbiFilename  wbiList=WBT_wbiList
  root_link : WBToolboxLibrary/wholeBodyModel/Kinematics/Forward Kinematics  frameName='root_link'  robotName=WBT_robotName  localName=WBT_modelName  wbiFile=WBT_wbiFilename  wbiList=WBT_wbiList
  w_H_root : Outport
  wires:
  Constant5/1 -> imu/1
  Inv\*/1 -> Inv\*2/1, holder 1/1, fromImuToHomogeousTransformFCN/1(imu_H_link)  "imu_H_link"
  imu/1 -> Inv\*/1
  Constant6/1 -> link/1
  Inv\*1/1 -> Switch6/3, fromImuToHomogeousTransformFCN/3(link_H_root)  "link_H_root"
  link/1 -> Inv\*/2, Inv\*1/1
  inertial/1 -> Selector/1, holder 2/1, fromImuToHomogeousTransformFCN/5(inertial)
  Switch6/1 -> w_H_root/1
  USE_IMU4EST_BASE/1 -> Switch6/2
  fromImuToHomogeousTransformFCN/1(w_H_root) -> Switch6/1
  Constant2/1 -> root_link/1
  qj/1 -> root_link/2, link/2, imu/2
  root_link/1 -> Inv\*1/2
  holder 1/1 -> fromImuToHomogeousTransformFCN/2(imu_H_link_0)
  holder 2/1 -> fromImuToHomogeousTransformFCN/4(inertial_0)
  Inv\*2/1 -> "CoM6D ->  CoMXYZ1"/1
  "CoM6D ->  CoMXYZ1"/1 -> Product/1  "l_sole_R_imu"
  Selector/1 -> Product/2  "imu_acce"
  Product/1 -> l_sole_acc/1
  Head state/1 -> Gain/1
  Selector1/1 -> Switch/1  "neck"
  USE_IMU4EST_BASE1/1 -> Switch/2
  Switch/1 -> fromImuToHomogeousTransformFCN/6(neck)
  Gain/1 -> Selector1/1
  Constant/1 -> Switch/3

== system torqueBalancingTuning/DesValues/State Machine/xCom ==
  qj : Inport
  w_H_b : Inport  Port=2
  "CoM6D ->  CoMXYZ2" : Selector  NumberOfDimensions=2  InputPortWidth=7  IndexOptions=Index vector (dialog),Index vector (dialog)  Indices=[1 2 3],[4]  OutputSizes=1,1
  com : WBToolboxLibrary/wholeBodyModel/Kinematics/Forward Kinematics  frameName='com'  robotName=WBT_robotName  localName=WBT_modelName  wbiFile=WBT_wbiFilename  wbiList=WBT_wbiList
  xCom : Outport
  wires:
  qj/1 -> com/2
  "CoM6D ->  CoMXYZ2"/1 -> xCom/1
  com/1 -> "CoM6D ->  CoMXYZ2"/1
  w_H_b/1 -> com/1

== system torqueBalancingTuning/DesValues/State Machine/xCom1 ==
  qj : Inport
  w_H_b : Inport  Port=2
  "CoM6D ->  CoMXYZ2" : Selector  NumberOfDimensions=2  InputPortWidth=7  IndexOptions=Index vector (dialog),Index vector (dialog)  Indices=[1 2 3],[4]  OutputSizes=1,1
  com : WBToolboxLibrary/wholeBodyModel/Kinematics/Forward Kinematics  frameName='com'  robotName=WBT_robotName  localName=WBT_modelName  wbiFile=WBT_wbiFilename  wbiList=WBT_wbiList
  xCom : Outport
  wires:
  qj/1 -> com/2
  "CoM6D ->  CoMXYZ2"/1 -> xCom/1
  com/1 -> "CoM6D ->  CoMXYZ2"/1
  w_H_b/1 -> com/1

== system torqueBalancingTuning/DesValues/State Machine Walking/Visualise extrnal wrenches   ==
  wL_WBDT : Inport
  wR_WBDT : Inport  Port=2
  Enable : EnablePort
  left foot ext wrench : Scope
  right foot ext wrench : Scope
  wires:
  wR_WBDT/1 -> right foot ext wrench/1  "wR_WBDT"
  wL_WBDT/1 -> left foot ext wrench/1  "wL_WBDT"

== system torqueBalancingTuning/DesValues/State Machine Walking/nu ==
  qj : Inport
  w_H_b : Inport  Port=2
  "constraints " : Inport  Port=3
  Get Estimate : WBToolboxLibrary/wholeBodyStates/Get Estimate  estimateType=Joints Velocity  robotName=WBT_robotName  localName=WBT_modelName  wbiFile=WBT_wbiFilename  wbiList=WBT_wbiList
  Jacobian l_sole : WBToolboxLibrary/wholeBodyModel/Jacobians/Jacobian  frameName='l_sole'  robotName=WBT_robotName  localName=WBT_modelName  wbiFile=WBT_wbiFilename  wbiList=WBT_wbiList
  Jacobian r_sole : WBToolboxLibrary/wholeBodyModel/Jacobians/Jacobian  frameName='r_sole'  robotName=WBT_robotName  localName=WBT_modelName  wbiFile=WBT_wbiFilename  wbiList=WBT_wbiList
  MATLAB Function : MATLAB Function  TreatAsAtomicUnit=on
  Mux : Mux  Inputs=2
  vb + Dqj : Outport
  wires:
  Get Estimate/1 -> MATLAB Function/4(qD), Mux/2
  Mux/1 -> vb + Dqj/1
  Jacobian r_sole/1 -> MATLAB Function/2(JcRightFoot)
  "constraints "/1 -> MATLAB Function/3(activeFeetConstraints)
  MATLAB Function/1(y) -> Mux/1
  Jacobian l_sole/1 -> MATLAB Function/1(JcLeftFoot)
  qj/1 -> Jacobian r_sole/2, Jacobian l_sole/2
  w_H_b/1 -> Jacobian r_sole/1, Jacobian l_sole/1

== system torqueBalancingTuning/DesValues/State Machine Walking/w_H_root_link1 ==
  qj : Inport
  inertial : Inport  Port=2
  "CoM6D ->  CoMXYZ1" : Selector  NumberOfDimensions=2  InputPortWidth=7  IndexOptions=Index vector (dialog),Index vector (dialog)  Indices=[1 2 3],[1 2 3]  OutputSizes=1,1
  Constant : Constant  Value=zeros(3,1)
  Constant2 : Constant  Value=eye(4)
  Constant5 : Constant  Value=eye(4)
  Constant6 : Constant  Value=eye(4)
  Gain : Gain  Gain=pi/180
  Head state : WBToolboxLibrary/Utilities/Yarp Read  portName=[WBT_robotName, '/head/state:o']  signalSize=6  blocking=off  timestamp=off  autoconnect=on  errorOnConnection=off
  Inv\* : Product  Inputs=/*  Multiplication=Matrix(*)
  Inv\*1 : Product  Inputs=/*  Multiplication=Matrix(*)
  Inv\*2 : Product  Inputs=/  Multiplication=Matrix(*)
  Product : Product  Multiplication=Matrix(*)
  Selector : Selector  InputPortWidth=12  IndexOptions=Index vector (dialog)  Indices=[4 5 6 ]  OutputSizes=1
  Selector1 : Selector  InputPortWidth=6  IndexOptions=Index vector (dialog)  Indices=[1:3]  OutputSizes=1
  Switch : Switch  Criteria=u2 > Threshold
  Switch6 : Switch  Criteria=u2 > Threshold
  USE_IMU4EST_BASE : Constant  Value=CONFIG.USE_IMU4EST_BASE
  USE_IMU4EST_BASE1 : Constant  Value=CONFIG.CORRECT_NECK_IMU
  fromImuToHomogeousTransformFCN : MATLAB Function  TreatAsAtomicUnit=on
  holder 1 : WBToolboxLibrary/Utilities/holder 
  holder 2 : WBToolboxLibrary/Utilities/holder 
  imu : WBToolboxLibrary/wholeBodyModel/Kinematics/Forward Kinematics  frameName='imu_frame'  robotName=WBT_robotName  localName=WBT_modelName  wbiFile=WBT_wbiFilename  wbiList=WBT_wbiList
  l_sole_acc : Scope
  link : WBToolboxLibrary/wholeBodyModel/Kinematics/Forward Kinematics  frameName=link_name  robotName=WBT_robotName  localName=WBT_modelName  wbiFile=WBT_wbiFilename  wbiList=WBT_wbiList
  root_link : WBToolboxLibrary/wholeBodyModel/Kinematics/Forward Kinematics  frameName='root_link'  robotName=WBT_robotName  localName=WBT_modelName  wbiFile=WBT_wbiFilename  wbiList=WBT_wbiList
  w_H_root : Outport
  wires:
  Constant5/1 -> imu/1
  Inv\*/1 -> Inv\*2/1, holder 1/1, fromImuToHomogeousTransformFCN/1(imu_H_link)  "imu_H_link"
  imu/1 -> Inv\*/1
  Constant6/1 -> link/1
  Inv\*1/1 -> Switch6/3, fromImuToHomogeousTransformFCN/3(link_H_root)  "link_H_root"
  link/1 -> Inv\*/2, Inv\*1/1
  inertial/1 -> Selector/1, holder 2/1, fromImuToHomogeousTransformFCN/5(inertial)
  Switch6/1 -> w_H_root/1
  USE_IMU4EST_BASE/1 -> Switch6/2
  fromImuToHomogeousTransformFCN/1(w_H_root) -> Switch6/1
  Constant2/1 -> root_link/1
  qj/1 -> root_link/2, link/2, imu/2
  root_link/1 -> Inv\*1/2
  holder 1/1 -> fromImuToHomogeousTransformFCN/2(imu_H_link_0)
  holder 2/1 -> fromImuToHomogeousTransformFCN/4(inertial_0)
  Inv\*2/1 -> "CoM6D ->  CoMXYZ1"/1
  "CoM6D ->  CoMXYZ1"/1 -> Product/1  "l_sole_R_imu"
  Selector/1 -> Product/2  "imu_acce"
  Product/1 -> l_sole_acc/1
  Head state/1 -> Gain/1
  Selector1/1 -> Switch/3  "neck"
  Constant/1 -> Switch/1
  USE_IMU4EST_BASE1/1 -> Switch/2
  Switch/1 -> fromImuToHomogeousTransformFCN/6(neck)
  Gain/1 -> Selector1/1

== system torqueBalancingTuning/DesValues/State Machine Walking/w_H_root_link4 ==
  qj : Inport
  inertial : Inport  Port=2
  "CoM6D ->  CoMXYZ1" : Selector  NumberOfDimensions=2  InputPortWidth=7  IndexOptions=Index vector (dialog),Index vector (dialog)  Indices=[1 2 3],[1 2 3]  OutputSizes=1,1
  Constant : Constant  Value=zeros(3,1)
  Constant2 : Constant  Value=eye(4)
  Constant5 : Constant  Value=eye(4)
  Constant6 : Constant  Value=eye(4)
  Gain : Gain  Gain=pi/180
  Head state : WBToolboxLibrary/Utilities/Yarp Read  portName=[WBT_robotName, '/head/state:o']  signalSize=6  blocking=off  timestamp=off  autoconnect=on  errorOnConnection=off
  Inv\* : Product  Inputs=/*  Multiplication=Matrix(*)
  Inv\*1 : Product  Inputs=/*  Multiplication=Matrix(*)
  Inv\*2 : Product  Inputs=/  Multiplication=Matrix(*)
  Product : Product  Multiplication=Matrix(*)
  Selector : Selector  InputPortWidth=12  IndexOptions=Index vector (dialog)  Indices=[4 5 6 ]  OutputSizes=1
  Selector1 : Selector  InputPortWidth=6  IndexOptions=Index vector (dialog)  Indices=[1:3]  OutputSizes=1
  Switch : Switch  Criteria=u2 > Threshold
  Switch6 : Switch  Criteria=u2 > Threshold
  USE_IMU4EST_BASE : Constant  Value=CONFIG.USE_IMU4EST_BASE
  USE_IMU4EST_BASE1 : Constant  Value=CONFIG.CORRECT_NECK_IMU
  fromImuToHomogeousTransformFCN : MATLAB Function  TreatAsAtomicUnit=on
  holder 1 : WBToolboxLibrary/Utilities/holder 
  holder 2 : WBToolboxLibrary/Utilities/holder 
  imu : WBToolboxLibrary/wholeBodyModel/Kinematics/Forward Kinematics  frameName='imu_frame'  robotName=WBT_robotName  localName=WBT_modelName  wbiFile=WBT_wbiFilename  wbiList=WBT_wbiList
  l_sole_acc : Scope
  link : WBToolboxLibrary/wholeBodyModel/Kinematics/Forward Kinematics  frameName=link_name  robotName=WBT_robotName  localName=WBT_modelName  wbiFile=WBT_wbiFilename  wbiList=WBT_wbiList
  root_link : WBToolboxLibrary/wholeBodyModel/Kinematics/Forward Kinematics  frameName='root_link'  robotName=WBT_robotName  localName=WBT_modelName  wbiFile=WBT_wbiFilename  wbiList=WBT_wbiList
  w_H_root : Outport
  wires:
  Constant5/1 -> imu/1
  Inv\*/1 -> Inv\*2/1, holder 1/1, fromImuToHomogeousTransformFCN/1(imu_H_link)  "imu_H_link"
  imu/1 -> Inv\*/1
  Constant6/1 -> link/1
  Inv\*1/1 -> Switch6/3, fromImuToHomogeousTransformFCN/3(link_H_root)  "link_H_root"
  link/1 -> Inv\*/2, Inv\*1/1
  inertial/1 -> Selector/1, holder 2/1, fromImuToHomogeousTransformFCN/5(inertial)
  Switch6/1 -> w_H_root/1
  USE_IMU4EST_BASE/1 -> Switch6/2
  fromImuToHomogeousTransformFCN/1(w_H_root) -> Switch6/1
  Constant2/1 -> root_link/1
  qj/1 -> root_link/2, link/2, imu/2
  root_link/1 -> Inv\*1/2
  holder 1/1 -> fromImuToHomogeousTransformFCN/2(imu_H_link_0)
  holder 2/1 -> fromImuToHomogeousTransformFCN/4(inertial_0)
  Inv\*2/1 -> "CoM6D ->  CoMXYZ1"/1
  "CoM6D ->  CoMXYZ1"/1 -> Product/1  "l_sole_R_imu"
  Selector/1 -> Product/2  "imu_acce"
  Product/1 -> l_sole_acc/1
  Head state/1 -> Gain/1
  Selector1/1 -> Switch/3  "neck"
  Constant/1 -> Switch/1
  USE_IMU4EST_BASE1/1 -> Switch/2
  Switch/1 -> fromImuToHomogeousTransformFCN/6(neck)
  Gain/1 -> Selector1/1

== system torqueBalancingTuning/DesValues/State Machine Walking/xCom ==
  qj : Inport
  w_H_b : Inport  Port=2
  "CoM6D ->  CoMXYZ2" : Selector  NumberOfDimensions=2  InputPortWidth=7  IndexOptions=Index vector (dialog),Index vector (dialog)  Indices=[1 2 3],[4]  OutputSizes=1,1
  com : WBToolboxLibrary/wholeBodyModel/Kinematics/Forward Kinematics  frameName='com'  robotName=WBT_robotName  localName=WBT_modelName  wbiFile=WBT_wbiFilename  wbiList=WBT_wbiList
  xCom : Outport
  wires:
  qj/1 -> com/2
  "CoM6D ->  CoMXYZ2"/1 -> xCom/1
  com/1 -> "CoM6D ->  CoMXYZ2"/1
  w_H_b/1 -> com/1

== system torqueBalancingTuning/DesValues/State Machine Walking/xCom1 ==
  qj : Inport
  w_H_b : Inport  Port=2
  "CoM6D ->  CoMXYZ2" : Selector  NumberOfDimensions=2  InputPortWidth=7  IndexOptions=Index vector (dialog),Index vector (dialog)  Indices=[1 2 3],[4]  OutputSizes=1,1
  com : WBToolboxLibrary/wholeBodyModel/Kinematics/Forward Kinematics  frameName='com'  robotName=WBT_robotName  localName=WBT_modelName  wbiFile=WBT_wbiFilename  wbiList=WBT_wbiList
  xCom : Outport
  wires:
  qj/1 -> com/2
  "CoM6D ->  CoMXYZ2"/1 -> xCom/1
  com/1 -> "CoM6D ->  CoMXYZ2"/1
  w_H_b/1 -> com/1

== system torqueBalancingTuning/controller_QP/QP/Visualize eventual QP failures ==
  exitFlagQP : Inport
  state : Inport  Port=2
  Enable : EnablePort
  "QP status (0: no failure, 1: not using)" : Scope  NumInputPorts=2
  wires:
  exitFlagQP/1 -> "QP status (0: no failure, 1: not using)"/1  "exitFlagQP"
  state/1 -> "QP status (0: no failure, 1: not using)"/2

== system torqueBalancingTuning/controller_QP/integralOf Hw1/w_H_root_link4 ==
  qj : Inport
  inertial : Inport  Port=2
  "CoM6D ->  CoMXYZ1" : Selector  NumberOfDimensions=2  InputPortWidth=7  IndexOptions=Index vector (dialog),Index vector (dialog)  Indices=[1 2 3],[1 2 3]  OutputSizes=1,1
  Constant : Constant  Value=zeros(3,1)
  Constant2 : Constant  Value=eye(4)
  Constant5 : Constant  Value=eye(4)
  Constant6 : Constant  Value=eye(4)
  Gain : Gain  Gain=pi/180
  Head state : WBToolboxLibrary/Utilities/Yarp Read  portName=[WBT_robotName, '/head/state:o']  signalSize=6  blocking=off  timestamp=off  autoconnect=on  errorOnConnection=off
  Inv\* : Product  Inputs=/*  Multiplication=Matrix(*)
  Inv\*1 : Product  Inputs=/*  Multiplication=Matrix(*)
  Inv\*2 : Product  Inputs=/  Multiplication=Matrix(*)
  Product : Product  Multiplication=Matrix(*)
  Selector : Selector  InputPortWidth=12  IndexOptions=Index vector (dialog)  Indices=[4 5 6 ]  OutputSizes=1
  Selector1 : Selector  InputPortWidth=6  IndexOptions=Index vector (dialog)  Indices=[1:3]  OutputSizes=1
  Switch : Switch  Criteria=u2 > Threshold
  Switch6 : Switch  Criteria=u2 > Threshold
  USE_IMU4EST_BASE : Constant  Value=CONFIG.USE_IMU4EST_BASE
  USE_IMU4EST_BASE1 : Constant  Value=CONFIG.CORRECT_NECK_IMU
  fromImuToHomogeousTransformFCN : MATLAB Function  TreatAsAtomicUnit=on
  holder 1 : WBToolboxLibrary/Utilities/holder 
  holder 2 : WBToolboxLibrary/Utilities/holder 
  imu : WBToolboxLibrary/wholeBodyModel/Kinematics/Forward Kinematics  frameName='imu_frame'  robotName=WBT_robotName  localName=WBT_modelName  wbiFile=WBT_wbiFilename  wbiList=WBT_wbiList
  l_sole_acc : Scope
  link : WBToolboxLibrary/wholeBodyModel/Kinematics/Forward Kinematics  frameName=link_name  robotName=WBT_robotName  localName=WBT_modelName  wbiFile=WBT_wbiFilename  wbiList=WBT_wbiList
  root_link : WBToolboxLibrary/wholeBodyModel/Kinematics/Forward Kinematics  frameName='root_link'  robotName=WBT_robotName  localName=WBT_modelName  wbiFile=WBT_wbiFilename  wbiList=WBT_wbiList
  w_H_root : Outport
  wires:
  Constant5/1 -> imu/1
  Inv\*/1 -> Inv\*2/1, holder 1/1, fromImuToHomogeousTransformFCN/1(imu_H_link)  "imu_H_link"
  imu/1 -> Inv\*/1
  Constant6/1 -> link/1
  Inv\*1/1 -> Switch6/3, fromImuToHomogeousTransformFCN/3(link_H_root)  "link_H_root"
  link/1 -> Inv\*/2, Inv\*1/1
  inertial/1 -> Selector/1, holder 2/1, fromImuToHomogeousTransformFCN/5(inertial)
  Switch6/1 -> w_H_root/1
  USE_IMU4EST_BASE/1 -> Switch6/2
  fromImuToHomogeousTransformFCN/1(w_H_root) -> Switch6/1
  Constant2/1 -> root_link/1
  qj/1 -> root_link/2, link/2, imu/2
  root_link/1 -> Inv\*1/2
  holder 1/1 -> fromImuToHomogeousTransformFCN/2(imu_H_link_0)
  holder 2/1 -> fromImuToHomogeousTransformFCN/4(inertial_0)
  Inv\*2/1 -> "CoM6D ->  CoMXYZ1"/1
  "CoM6D ->  CoMXYZ1"/1 -> Product/1  "l_sole_R_imu"
  Selector/1 -> Product/2  "imu_acce"
  Product/1 -> l_sole_acc/1
  Head state/1 -> Gain/1
  Selector1/1 -> Switch/3  "neck"
  Constant/1 -> Switch/1
  USE_IMU4EST_BASE1/1 -> Switch/2
  Switch/1 -> fromImuToHomogeousTransformFCN/6(neck)
  Gain/1 -> Selector1/1

== system torqueBalancingTuning/DesValues/LinearizationAndGainTuning/Subsystem/centroidalMomentumMatrix ==
  W_H_b : Inport
  qj : Inport  Port=2
  JGbase : Subsystem
  JGjoints : Subsystem
  Matrix Concatenate : Concatenate  Mode=Multidimensional array  ConcatenateDimension=2
  JG : Outport
  wires:
  qj/1 -> JGjoints/1(qj), JGbase/1(qj)
  W_H_b/1 -> JGjoints/2(W_H_b), JGbase/2(W_H_b)
  JGbase/1(JGbase) -> Matrix Concatenate/1
  JGjoints/1(JGjoints) -> Matrix Concatenate/2
  Matrix Concatenate/1 -> JG/1
